simulink model "Motor"  (R2015b)
settings: Solver=FixedStepAuto  StartTime=0.0  StopTime=10.0  FixedStep=0.1  RelTol=1e-3
settings Model: Creator=Deepak  LastModifiedBy=Deepak

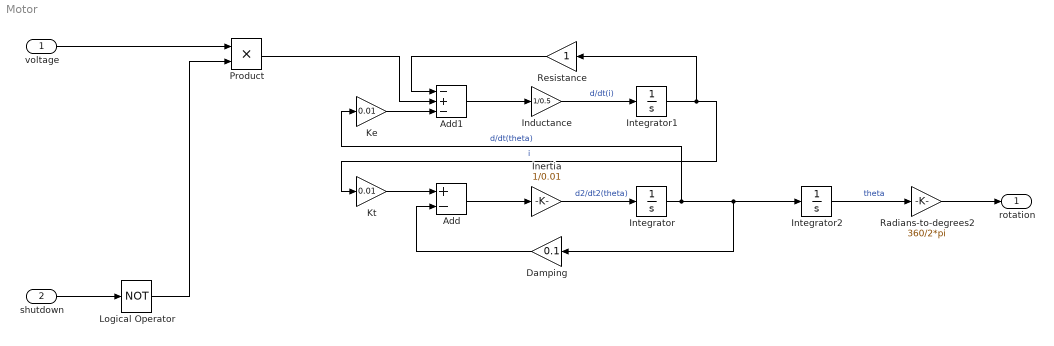
== system Motor ==
  voltage : Inport
  shutdown : Inport  Port=2
  Add : Sum  Inputs=+-
  Add1 : Sum  Inputs=-+-
  Damping : Gain  Gain=0.1
  Inductance : Gain  Gain=1/0.5
  Inertia : Gain  Gain=1/0.01
  Integrator : Integrator
  Integrator1 : Integrator
  Integrator2 : Integrator
  Ke : Gain  Gain=0.01
  Kt : Gain  Gain=0.01
  Logical Operator : Logic  Operator=NOT  AllPortsSameDT=off  OutDataTypeStr=boolean
  Product : Product
  Radians-to-degrees2 : Gain  Gain=360/2*pi
  Resistance : Gain
  rotation : Outport
      settings: AttributesFormatString=angle
  wires:
  Integrator1/1 -> Kt/1, Resistance/1  "i"
  Inductance/1 -> Integrator1/1  "d/dt(i)"
  Inertia/1 -> Integrator/1  "d2/dt2(theta)"
  Integrator/1 -> Ke/1, Integrator2/1, Damping/1  "d/dt(theta)"
  Add1/1 -> Inductance/1
  Add/1 -> Inertia/1
  Damping/1 -> Add/2
  Kt/1 -> Add/1
  Resistance/1 -> Add1/1
  Ke/1 -> Add1/3
  Product/1 -> Add1/2
  Logical Operator/1 -> Product/2
  Integrator2/1 -> Radians-to-degrees2/1  "theta"
  shutdown/1 -> Logical Operator/1
  voltage/1 -> Product/1
  Radians-to-degrees2/1 -> rotation/1
